simulink model "sldemo_mdlref_heat2cost"  (Simulink 7.6)
settings: Solver=ode3  SolverMode=SingleTasking  StartTime=0.0  StopTime=2*24*60*60  FixedStep=60  RelTol=1e-3  AbsTol=1e-6
model workspace (MAT data in the model file):
  cost : num (value not decoded)
settings Model: Creator=The MathWorks Inc.  ExtModeAutoUpdateStatusClock=off
settings DataIOCC: ExternalInput=[]  InitialState=[]  LimitDataPoints=off  SaveOutput=off  SaveTime=off
settings OptimizationCC: BlockReduction=off  BooleanDataType=off  InlineParams=on  InlineInvariantSignals=on  InitFltsAndDblsToZero=on
settings DebuggingCC: SaveWithParameterizedLinksMsg=none  CheckExecutionContextPreStartOutputMsg=on  CheckExecutionContextRuntimeOutputMsg=on  SolverPrmCheckMsg=none  MultiTaskDSMMsg=warning  MultiTaskCondExecSysMsg=none  SigSpecEnsureSampleTimeMsg=none  IntegerOverflowMsg=none
settings RTWCC: IncludeERTFirstTime=on
settings CodeAppCC: MaxIdLength=100
settings GRTTargetCC: TargetFcnLib=ansi_tfl_tmw.mat

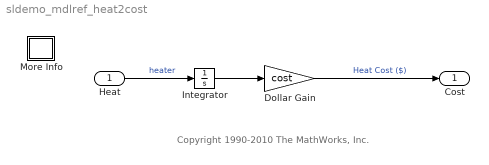
== system sldemo_mdlref_heat2cost ==
  note: Copyright 1990-2010 The MathWorks, Inc.
  Heat : Inport  OutDataTypeStr=double  PortDimensions=1  SampleTime=0
  Dollar Gain : Gain  Gain=cost  SaturateOnIntegerOverflow=on  OutDataTypeStr=Inherit: Same as input  ParamDataTypeStr=Inherit: Same as input
  Integrator : Integrator
  More Info : Subsystem
      settings: OpenFcn=showdemo('sldemo_mdlref_depgraph')
      mask Display: disp('?')
  Cost : Outport
  wires:
  Dollar Gain/1 -> Cost/1  "Heat Cost ($)"
  Heat/1 -> Integrator/1  "heater"
  Integrator/1 -> Dollar Gain/1

== system sldemo_mdlref_heat2cost/More Info ==
